simulink model "Beobachter"  (R2020a)
settings: Solver=ode8  StartTime=0.0  StopTime=10.0  RelTol=1e-3
model workspace (MAT data in the model file):
  A = Simulink.Parameter
  A.Value = [0  1; 0  0]
  A.DataType = 'auto'
  A.Complexity = 'real'
  A.Dimensions = [2 2]
  B = Simulink.Parameter
  B.Value = [0; 7.007]
  B.DataType = 'auto'
  B.Complexity = 'real'
  B.Dimensions = [2 1]
  C = Simulink.Parameter
  C.Value = [1 0]
  C.DataType = 'auto'
  C.Complexity = 'real'
  C.Dimensions = [1 2]
  K = Simulink.Parameter
  K.Value = [0.4281 0.5708]
  K.DataType = 'auto'
  K.Complexity = 'real'
  K.Dimensions = [1 2]
  L = Simulink.Parameter
  L.Value = [40 300]
  L.DataType = 'auto'
  L.Complexity = 'real'
  L.Dimensions = [1 2]
settings Model: ParameterArgumentNames=K  Creator=Hoorsana  LastModifiedBy=Hoorsana
settings DebuggingCC: SFMachineParentedDataDiag=error

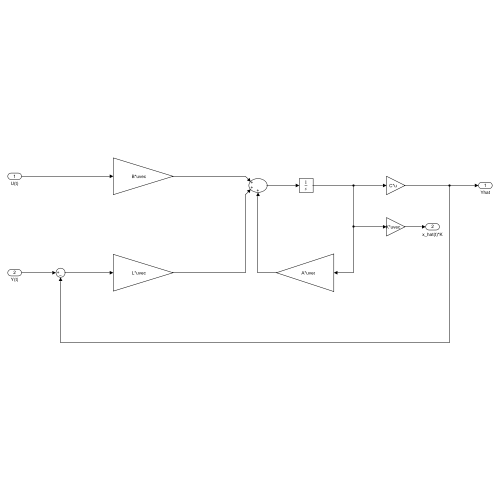
[thumbnail: Simulink's stored preview of the top-level diagram]
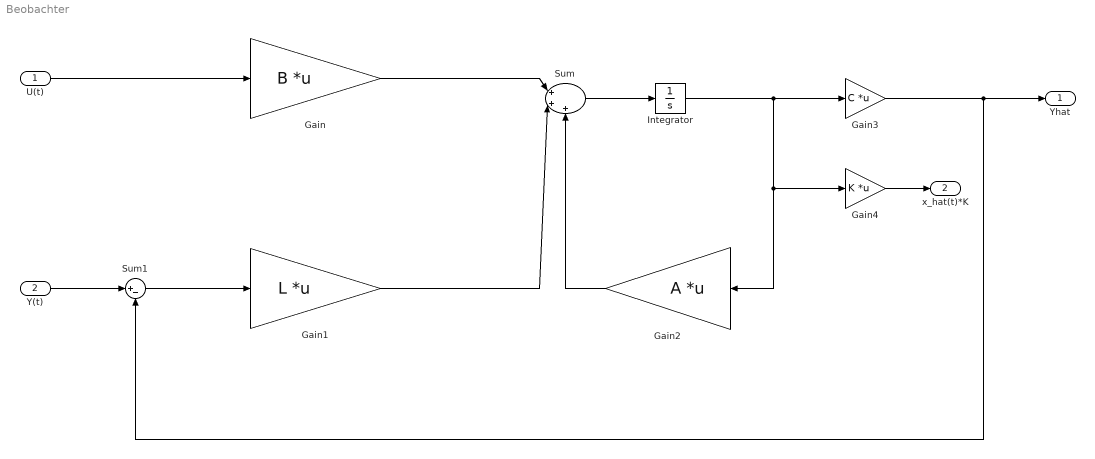
== system Beobachter ==
  U(t) : Inport
  Y(t) : Inport  Port=2
  Gain : Gain  Gain=B  Multiplication=Matrix(K*u) (u vector)
  Gain1 : Gain  Gain=L  Multiplication=Matrix(K*u) (u vector)
  Gain2 : Gain  Gain=A  Multiplication=Matrix(K*u) (u vector)
  Gain3 : Gain  Gain=C  Multiplication=Matrix(K*u)
  Gain4 : Gain  Gain=K  Multiplication=Matrix(K*u) (u vector)
  Integrator : Integrator
  Sum : Sum  Inputs=|+++
  Sum1 : Sum  Inputs=|+-
  Yhat : Outport
  x_hat(t)*K : Outport  Port=2  VectorParamsAs1DForOutWhenUnconnected=off
  wires:
  Sum1/1 -> Gain1/1
  Gain1/1 -> Sum/2
  Integrator/1 -> Gain2/1, Gain4/1, Gain3/1
  Gain2/1 -> Sum/3
  Sum/1 -> Integrator/1
  Gain4/1 -> x_hat(t)*K/1
  Gain/1 -> Sum/1
  Gain3/1 -> Sum1/2, Yhat/1
  Y(t)/1 -> Sum1/1
  U(t)/1 -> Gain/1
